simulink model "WheelSizing"  (R2023a)
settings: Solver=VariableStepAuto  StartTime=0.0  StopTime=6000  RelTol=1e-8
values from neighbouring files (symbols this model uses):
  euler_b_LVLH = [atan2(M(2,3),M(3,3)); -asin(M(1,3)); atan2(M(1,2),M(1,1))]    [A421_FinalProj_MainScript.m]    (also in WheelSizing_Script.m)
  I_ReactionWheels = J.normal + (2 * It + Is + 2 * mw) * eye(3)    [WheelSizing_Script.m]
  kd = 2 * zeta * wn .* J.normal    [WheelSizing_Script.m]
  kp = wn^2 * 2 .* J.normal    [WheelSizing_Script.m]
  qc = [0;0;0;1]    [WheelSizing_Script.m]
  r_ECI = Qperi2geo*r_PF    [WheelSizing_Script.m]
  rv_initial = [r_ECI;v_ECI]    [A421_FinalProj_MainScript.m]    (also in WheelSizing_Script.m)
  sun_ECI = [1; 0; 0]    [WheelSizing_Script.m]
  surfaceProperties = [Areas cps normals]    [WheelSizing_Script.m]
  v_ECI = Qperi2geo*v_PF    [WheelSizing_Script.m]
undefined symbols (not defined in the file or in its folder): J, normal
settings Model: Creator=jself  LastModifiedBy=willb
settings DebuggingCC: UnconnectedInputMsg=warning  UnconnectedOutputMsg=warning  UnconnectedLineMsg=warning
settings ModelReferenceCC: EnableRefExpFcnMdlSchedulingChecks=on
settings RTWCC: DLArmComputeVersion=19.05

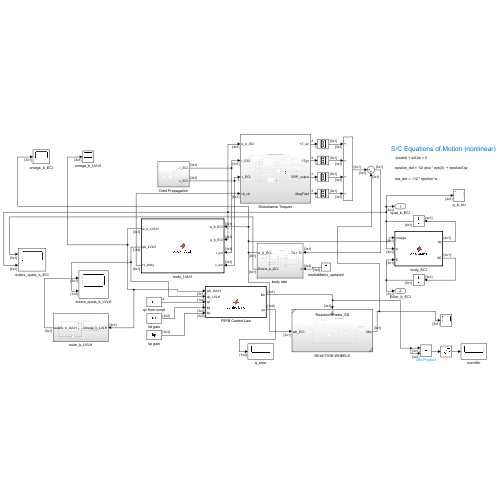
[thumbnail: Simulink's stored preview of the top-level diagram]
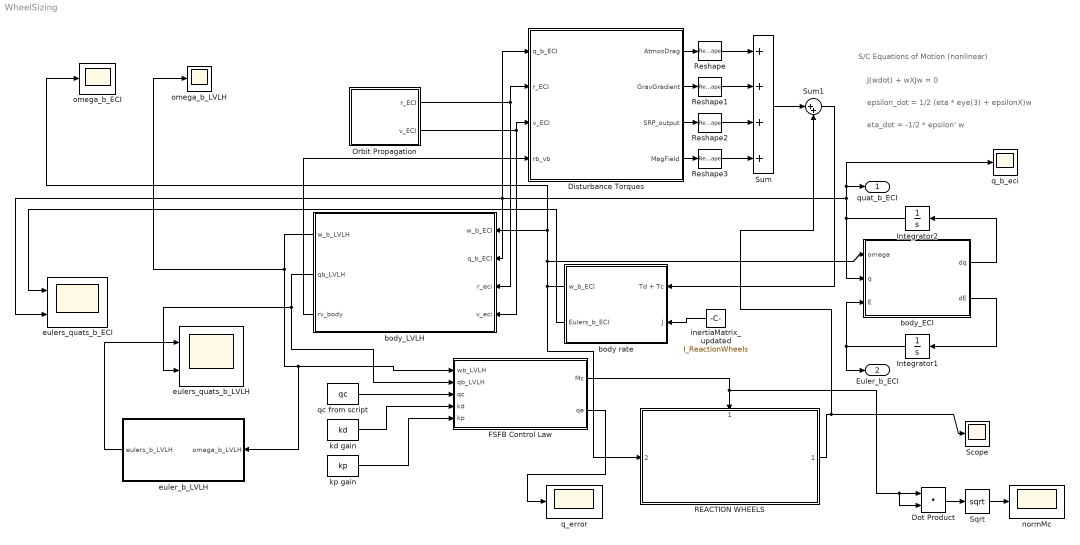
== system WheelSizing ==
  note: eta_dot = -1/2 * epsilon' w
  note: epsilon_dot = 1/2 (eta * eye(3) + epsilonX)w
  note: J(wdot) + wXJw = 0
  note: S/C Equations of Motion (nonlinear)
  Disturbance Torques : Subsystem
  Dot Product : DotProduct  OutDataTypeStr=Inherit: Inherit via internal rule
  FSFB Control Law : MATLAB Function  TreatAsAtomicUnit=on
  Integrator1 : Integrator  InitialCondition=normal.state(4:6)
  Integrator2 : Integrator  InitialCondition=normal.state(7:10)
  Orbit Propagation : Subsystem
  REACTION WHEELS : Subsystem  ReferencedSubsystem=ReactionWheels_SS
      settings: PortSchema="{\"entries\":[{\"content\":{\"sides\":[{\"content\":{\"connectorIds\":[\"In2\"]},\"type\":\"ConnectorPlacement.EquallySpacedRectSide\",\"uuid\":\"17b22d00-74c7-41dc-9281-1170939ab431\"},{\"content\":{\"connectorIds\":[\"Out1\"],\"side\":\"RIGHT\"},\"type\":\"ConnectorPlacement.EquallySpacedRectSide\",\"uuid\":\"47f34f04-9630-46fb-894e-c63a456fb1f8\"},{\"content\":{\"connectorIds\":[\"In1\"],\"side\":\"TOP\"},\"type\":\"ConnectorPlacement.EquallySpacedRectSide\",\"uuid\":\"0e15db1d-4c6b-4e54-83e4-cf923cd0db41\"}]},\"type\":\"ConnectorPlacement.EquallySpacedConnector\",\"uuid\":\"f035ae7b-0a11-467c-88f1-219b3350dd2e\"}],\"packageUris\":[\"http://schema.mathworks.com/mf0/Connector/R2020b\"],\"version\":\"1.0\"}"
  Reshape{,1..3} (4 alike) : Reshape  OutputDimensionality=Column vector (2-D)
  Scope : Scope
  Sqrt : Sqrt
  Sum : Sum  Inputs=++++
  Sum1 : Sum  Inputs=|++
  "body rate " : Subsystem
  body_ECI : MATLAB Function  TreatAsAtomicUnit=on
  body_LVLH : MATLAB Function  TreatAsAtomicUnit=on
  euler_b_LVLH : Subsystem
  eulers_quats_b_ECI : Scope  NumInputPorts=2
  eulers_quats_b_LVLH : Scope  NumInputPorts=2
  inertiaMatrix_updated : Constant  Value=I_ReactionWheels
  kd gain : Constant  Value=kd
  kp gain : Constant  Value=kp
  normMc : Scope
  omega_b_ECI : Scope
  omega_b_LVLH : Scope
  q_b_eci : Scope
  q_error : Scope
  qc from script : Constant  Value=qc
  quat_b_ECI : Outport  PortDimensions=[4 1]
  Euler_b_ECI : Outport  Port=2  PortDimensions=[3 1]
  wires:
  inertiaMatrix_updated/1 -> "body rate "/2(J)
  Disturbance Torques/1(AtmosDrag) -> Reshape/1
  Disturbance Torques/3(SRP_output) -> Reshape2/1
  body_LVLH/1(w_b_LVLH) -> omega_b_LVLH/1, euler_b_LVLH/1(omega_b_LVLH), FSFB Control Law/1(wb_LVLH)
  Orbit Propagation/1(r_ECI) -> body_LVLH/3(r_eci), Disturbance Torques/2(r_ECI)
  Orbit Propagation/2(v_ECI) -> Disturbance Torques/3(v_ECI), body_LVLH/4(v_eci)
  Sum1/1 -> "body rate "/1(Td + Tc)
  body_ECI/2(dE) -> Integrator1/1
  Integrator1/1 -> Euler_b_ECI/1, body_ECI/3(E)
  body_ECI/1(dq) -> Integrator2/1
  "body rate "/1(w_b_ECI) -> REACTION WHEELS/2, body_LVLH/1(w_b_ECI), omega_b_ECI/1, body_ECI/1(omega)
  kp gain/1 -> FSFB Control Law/5(kp)
  kd gain/1 -> FSFB Control Law/4(kd)
  qc from script/1 -> FSFB Control Law/3(qc)
  body_LVLH/2(qb_LVLH) -> eulers_quats_b_LVLH/2, FSFB Control Law/2(qb_LVLH)
  Integrator2/1 -> Disturbance Torques/1(q_b_ECI), eulers_quats_b_ECI/2, body_LVLH/2(q_b_ECI), q_b_eci/1, quat_b_ECI/1, body_ECI/2(q)
  body_LVLH/3(rv_body) -> Disturbance Torques/4(rb_vb)
  FSFB Control Law/2(qe) -> q_error/1
  FSFB Control Law/1(Mc) -> Dot Product/2, Dot Product/1, REACTION WHEELS/1
  Sum/1 -> Sum1/1
  Reshape/1 -> Sum/1
  Disturbance Torques/4(MagField) -> Reshape3/1
  Reshape3/1 -> Sum/4
  Reshape2/1 -> Sum/3
  Disturbance Torques/2(GravGradient) -> Reshape1/1
  Reshape1/1 -> Sum/2
  "body rate "/2(Eulers_b_ECI) -> eulers_quats_b_ECI/1
  euler_b_LVLH/1(eulers_b_LVLH) -> eulers_quats_b_LVLH/1
  REACTION WHEELS/1 -> Sum1/2, Scope/1
  Sqrt/1 -> normMc/1
  Dot Product/1 -> Sqrt/1

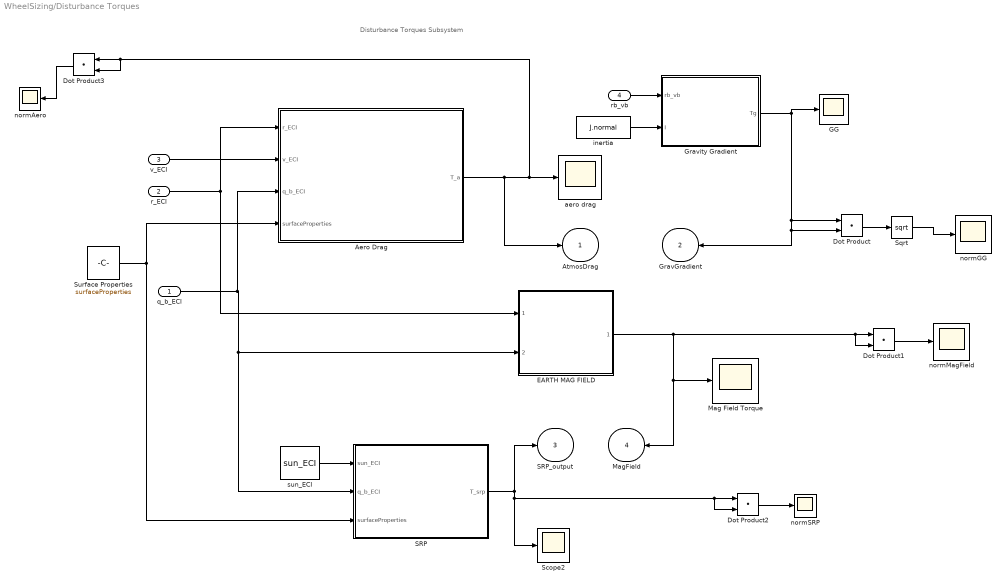
== system WheelSizing/Disturbance Torques ==
  note: Disturbance Torques Subsystem
  q_b_ECI : Inport  PortDimensions=[4 1]
  r_ECI : Inport  Port=2
  v_ECI : Inport  Port=3  PortDimensions=3
  rb_vb : Inport  Port=4
  Aero Drag : MATLAB Function  TreatAsAtomicUnit=on
  Dot Product{,1..3} (4 alike) : DotProduct  OutDataTypeStr=Inherit: Inherit via internal rule
  EARTH MAG FIELD : Subsystem  ReferencedSubsystem=EarthMagneticField_SS
  GG : Scope
  Gravity Gradient : MATLAB Function  TreatAsAtomicUnit=on
  Mag Field Torque : Scope
  SRP : MATLAB Function  TreatAsAtomicUnit=on
  Scope2 : Scope
  Sqrt : Sqrt
  Surface Properties : Constant  Value=surfaceProperties
  aero drag : Scope
  inertia : Constant  Value=J.normal
  normAero : Scope
  normGG : Scope
  normMagField : Scope
  normSRP : Scope
  sun_ECI : Constant  Value=sun_ECI
  AtmosDrag : Outport
  GravGradient : Outport  Port=2
  SRP_output : Outport  Port=3
  MagField : Outport  Port=4
  wires:
  Gravity Gradient/1(Tg) -> GG/1, Dot Product/1, Dot Product/2, GravGradient/1
  SRP/1(T_srp) -> Scope2/1, Dot Product2/2, Dot Product2/1, SRP_output/1
  Aero Drag/1(T_a) -> Dot Product3/2, Dot Product3/1, aero drag/1, AtmosDrag/1
  sun_ECI/1 -> SRP/1(sun_ECI)
  v_ECI/1 -> Aero Drag/2(v_ECI)
  q_b_ECI/1 -> SRP/2(q_b_ECI), EARTH MAG FIELD/2, Aero Drag/3(q_b_ECI)
  r_ECI/1 -> EARTH MAG FIELD/1, Aero Drag/1(r_ECI)
  EARTH MAG FIELD/1 -> MagField/1, Mag Field Torque/1, Dot Product1/2, Dot Product1/1
  Surface Properties/1 -> SRP/3(surfaceProperties), Aero Drag/4(surfaceProperties)
  rb_vb/1 -> Gravity Gradient/1(rb_vb)
  inertia/1 -> Gravity Gradient/2(I)
  Dot Product/1 -> Sqrt/1
  Sqrt/1 -> normGG/1
  Dot Product1/1 -> normMagField/1
  Dot Product2/1 -> normSRP/1
  Dot Product3/1 -> normAero/1

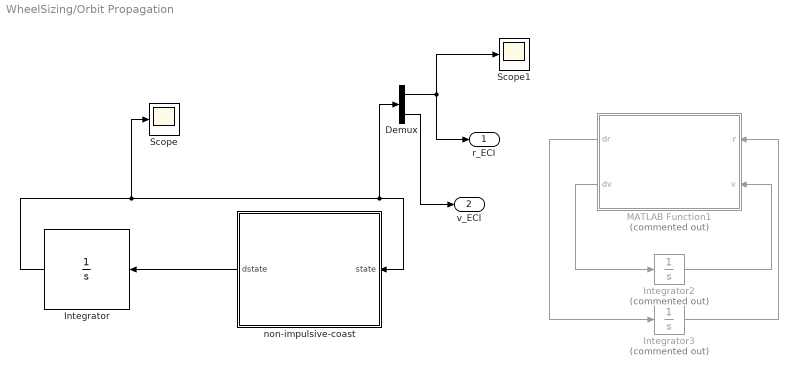
== system WheelSizing/Orbit Propagation ==
  Demux : Demux  Outputs=2
  Integrator : Integrator  InitialCondition=rv_initial
  Integrator2 : Integrator  Commented=on  InitialCondition=r_ECI
  Integrator3 : Integrator  Commented=on  InitialCondition=v_ECI
  MATLAB Function1 : MATLAB Function  Commented=on  TreatAsAtomicUnit=on
  Scope : Scope
  Scope1 : Scope
  non-impulsive-coast : MATLAB Function  TreatAsAtomicUnit=on
  r_ECI : Outport  PortDimensions=[3 1]  VectorParamsAs1DForOutWhenUnconnected=off
  v_ECI : Outport  Port=2  PortDimensions=[3 1]  VectorParamsAs1DForOutWhenUnconnected=off
  wires:
  Integrator2/1 -> MATLAB Function1/2(v)
  MATLAB Function1/1(dr) -> Integrator3/1
  MATLAB Function1/2(dv) -> Integrator2/1
  Integrator3/1 -> MATLAB Function1/1(r)
  non-impulsive-coast/1(dstate) -> Integrator/1
  Integrator/1 -> Scope/1, Demux/1, non-impulsive-coast/1(state)
  Demux/1 -> Scope1/1, r_ECI/1
  Demux/2 -> v_ECI/1

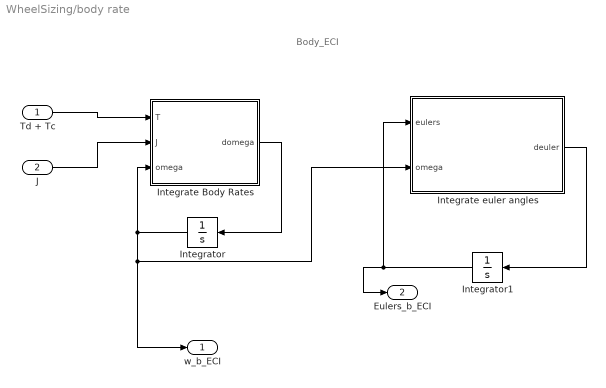
== system WheelSizing/body rate  ==
  note: Body_ECI
  Td + Tc : Inport
  J : Inport  Port=2
  Integrate Body Rates : MATLAB Function  TreatAsAtomicUnit=on
  Integrate euler angles : MATLAB Function  TreatAsAtomicUnit=on
  Integrator : Integrator  InitialCondition=normal.state(1:3)
  Integrator1 : Integrator  InitialCondition=normal.state(4:6)
  w_b_ECI : Outport  PortDimensions=[3 1]
  Eulers_b_ECI : Outport  Port=2
  wires:
  J/1 -> Integrate Body Rates/2(J)
  Td + Tc/1 -> Integrate Body Rates/1(T)
  Integrate Body Rates/1(domega) -> Integrator/1
  Integrator/1 -> Integrate euler angles/2(omega), w_b_ECI/1, Integrate Body Rates/3(omega)
  Integrate euler angles/1(deuler) -> Integrator1/1
  Integrator1/1 -> Eulers_b_ECI/1, Integrate euler angles/1(eulers)

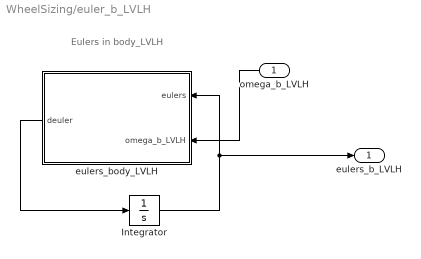
== system WheelSizing/euler_b_LVLH ==
  note: Eulers in body_LVLH
  omega_b_LVLH : Inport
  Integrator : Integrator  InitialCondition=euler_b_LVLH
  eulers_body_LVLH : MATLAB Function  TreatAsAtomicUnit=on
  eulers_b_LVLH : Outport
  wires:
  eulers_body_LVLH/1(deuler) -> Integrator/1
  Integrator/1 -> eulers_b_LVLH/1, eulers_body_LVLH/1(eulers)
  omega_b_LVLH/1 -> eulers_body_LVLH/2(omega_b_LVLH)

== matlab function WheelSizing/Disturbance Torques/Aero Drag ==
  data: r_ECI input; v_ECI input; T_a output; q_b_ECI input; surfaceProperties input
function T_a = aero_drag_torque(r_ECI, v_ECI, q_b_ECI, surfaceProperties) 


q_b_ECI = q_b_ECI'; 
q_b_ECI = [q_b_ECI(4), q_b_ECI(1), q_b_ECI(2), q_b_ECI(3)]; 
v_b = quat2rotm(q_b_ECI)*v_ECI;
Cd = 2.1;
Re = 6378.137;

rho_0 = 3.614e-14;
H = 88.667;
h_0 = 700;
density = rho_0*exp(-(norm(r_ECI) - Re - h_0)/H);
T_a = zeros([3,1]);

for i = 1:length(surfaceProperties)
    A = surfaceProperties(i,1);
    cp = surfaceProperties(i,2:4);
    n = surfaceProperties(i,5:7);
    wet = n*v_b/norm(v_b);
    if wet > 0
        A_wet = A*wet;
        v_b_hat = v_b/norm(v_b);
        F_a = -1/2*density*(norm(v_ECI)*1000)^2*Cd*A_wet*v_b_hat;
        T_a = T_a + cross(cp', F_a);
    end
end

== matlab function WheelSizing/FSFB Control Law ==
  data: wb_LVLH input; qb_LVLH input; qc input; Mc output; kd input; kp input; qe output
% this is JUSTIN'S gain selection code from an old assignment

function [Mc,qe]  = controlLaw(wb_LVLH, qb_LVLH, qc, kd, kp)

% Torque output goes to equations of motion
% epsilon error only ouputting to verify that it converges to 0. 

qc = [qc(4),qc(1),qc(2),qc(3)]; % ROW; ETA FIRST

% MODIFYING INPUTS; quaternion only
% 1. ROW VECTOR
% 2. ETA FIRST, THEN EPSILON for all MATLAB quat functions

q = qb_LVLH; % row; ETA FIRST 
w = wb_LVLH; 

% We give up and create our functions...
qe = quatMult(quatConj(qc),q);
% out == eta first; row
% qe = [qe(4),qe(1),qe(2),qe(3)]; % now ETA IS FIRST

Epsilon_error = qe(2:4); % row; eta first.

% Control law
Mc = -kp*Epsilon_error' - kd*w;
 
end

== matlab function WheelSizing/body rate /Integrate euler angles ==
  data: eulers input; deuler output; omega input
function deuler = euler_rates(eulers,omega)

% Euler Angles
phi = eulers(1);
theta = eulers(2);
psi = eulers(3);

deuler = cos(theta)^(-1) * [   cos(theta)      sin(phi)*sin(theta)     cos(phi)*sin(theta); 
                                0               cos(phi)*cos(theta)     -sin(phi)*cos(theta);
                                0               sin(phi)                 cos(phi)           ] * omega;

== matlab function WheelSizing/body_LVLH ==
  data: w_b_ECI input; q_b_ECI input; r_eci input; v_eci input; w_b_LVLH output; qb_LVLH output; rv_body output
function [w_b_LVLH, qb_LVLH, rv_body] = body_LVLH(w_b_ECI, q_b_ECI, r_eci, v_eci)

% ASSUME ETA COMES IN FIRST
% epsilon_ECI = q_b_ECI(2:4); 
% eta_ECI = q_b_ECI(1); 
epsilon_ECI = q_b_ECI(1:3); 
eta_ECI = q_b_ECI(4);


[Cb_ECI] = quat2rotationmatrix(epsilon_ECI,eta_ECI); 

w_LVLH_ECI = (cross(r_eci,v_eci))/(norm(r_eci)^2);  
w_b_LVLH = w_b_ECI - Cb_ECI*w_LVLH_ECI; 

% ECI to LVLH for getting q_b_LVLH 
rmag_eci = norm(r_eci);                                                     
h_eci = cross(r_eci,v_eci);
hmag_eci = norm(h_eci);

% ECI to LVLH
z = -r_eci/rmag_eci;
y = -h_eci/hmag_eci;
x = cross(y,z);
C_LVLH_ECI = [x'; y'; z'];

% Get Cb_LVLH
Cb_LVLH = Cb_ECI * C_LVLH_ECI'; 

% Get qb_LVLH 
qb_LVLH = C2quat_altVersion(Cb_LVLH); % ROW VECTOR; eta first 
%qb_LVLH = C2quat(Cb_LVLH); %eta first

rv_body = [Cb_ECI * r_eci; Cb_ECI * v_eci]; 


end

== matlab function WheelSizing/euler_b_LVLH/eulers_body_LVLH ==
  data: eulers input; deuler output; omega_b_LVLH input
function deuler = euler_rates(eulers,omega_b_LVLH)

% Euler Angles

phi = eulers(1);
theta = eulers(2);
psi = eulers(3);

deuler = cos(theta)^(-1) * [   cos(theta)      sin(phi)*sin(theta)     cos(phi)*sin(theta); 
                                0               cos(phi)*cos(theta)     -sin(phi)*cos(theta);
                                0               sin(phi)                 cos(phi)           ] * omega_b_LVLH;

== matlab function WheelSizing/Orbit Propagation/MATLAB Function1 ==
  data: r input; dr output; v input; dv output
function [dr,dv] = orbitalDynamic(r,v)

mu = 398600; 

dr = v; 
dv = -mu*r/norm(r); 

end

== matlab function WheelSizing/body rate /Integrate Body Rates ==
  data: T input; domega output; J input; omega input
function domega  = dynamics(T, J, omega)

domega = J\(T - cross(omega, J*omega)); 

end

== matlab function WheelSizing/Orbit Propagation/non-impulsive-coast ==
  data: state input; dstate output
function dstate = non_impulsive_COAST(state)
%{ 

*FOR COAST PHASE ONLY*

**This function assumes that thrust is exactly parallel to initial velocity
direction.

This function is for numerical integration (i.e., plug into ode45).
NOTE: only use this function for the BURN PHASE of the non-impulsive
maneuver. For the BURN phase, use "non_impulsive_BURN"

INPUTS: 
    INITIAL CONDITIONS
    state vector(1:3) = position (rx,ry,rz)
    state vector(4:6) = velocity (vx,vy,vz)

OUTPUT: New state vector after integration.
%%%%%%%%%%%%%%%%%%%%%%%%%%%%%%%%%%%%%%%%%%%%%%%%%
Justin Self, Cal Poly, Fall 2022; Introduction to Orbital Mechanics.
%%%%%%%%%%%%%%%%%%%%%%%%%%%%%%%%%%%%%%%%%%%%%%%%%
%}

mu = 398600;

rx = state(1);
ry = state(2);
rz = state(3);
vx = state(4);
vy = state(5);
vz = state(6);

r_vect = [rx ry rz];
r = norm(r_vect);

v_vect = [vx vy vz];
v = norm(v_vect);

xdot = vx;
ydot = vy;
zdot = vz;
xddot = (-mu*rx)/(r^3);
yddot = (-mu*ry)/(r^3);
zddot = (-mu*rz)/(r^3);

dstate = [xdot; ydot; zdot; xddot; yddot; zddot];

% rState = dstate(1:3);
% vState = dstate(4:6);

end

== matlab function WheelSizing/body_ECI ==
  data: omega input; dq output; q input; E input; dE output
function [dq,dE] = kinematics(omega, q, E)


% unpack quaternion
% epsilon = q(1:3,1);
% eta = q(4,1);
% depsilon = 1/2*(eta*eye(3) + vect2cross(epsilon))*omega;
% deta = -1/2*epsilon'*omega;
% dq = [depsilon; deta];

epx = q(1);
epy = q(2);
epz = q(3);
eta = q(4);
epsilon = [epx; epy; epz];
epsilon_cross = [   0       -epz     epy;
                    epz     0        -epx;
                    -epy    epx      0    ];

% Derivatives of epsilon and eta
depsilon = 0.5 * (eta*eye(3) + epsilon_cross) * omega;
deta = -0.5 * epsilon' * omega;
dq = [depsilon(1); depsilon(2); depsilon(3); deta]; % ETA LAST

% Euler Angle 
LBI = 1/cos(E(2))*[cos(E(2)) sin(E(1))*sin(E(2))  cos(E(1))*sin(E(2));
                   0         cos(E(1))*cos(E(2)) -sin(E(1))*cos(E(2));
                   0         sin(E(1))            cos(E(1))];
dE = LBI*omega;

end

== matlab function WheelSizing/Disturbance Torques/SRP ==
  data: sun_ECI input; T_srp output; q_b_ECI input; surfaceProperties input
function T_srp  = SPR_torque(sun_ECI, q_b_ECI, surfaceProperties)

p_sun = 4.5e-6; %N/m
q_b_ECI = q_b_ECI'; 
q_b_ECI = [q_b_ECI(4), q_b_ECI(1), q_b_ECI(2), q_b_ECI(3)]; 

sun_b = quat2rotm(q_b_ECI) * sun_ECI;
T_srp = zeros([3,1]);
%rho_sum = zeros([3,1]);
% Solar Radiation Pressure
for i = 1:length(surfaceProperties)
    A = surfaceProperties(i,1);
    cp = surfaceProperties(i,2:4);
    n = surfaceProperties(i,5:7);
    wet = n*sun_b/norm(sun_b);
    if wet > 0
        A_wet = A*wet;
        F_srp = p_sun*A_wet*sun_b;
        T_srp = T_srp + cross(cp', F_srp);
        %rho_sum = rho_sum + rho';
    end
end

== matlab function WheelSizing/Disturbance Torques/Gravity Gradient ==
  data: rb_vb input; Tg output; I input
% function T_gg = gg_torque(r_ECI, q_b_ECI, J)
% 
% mu = 398600;
% 
% % R in body
% r_b = quat2rotm(q_b_ECI)*r_ECI;
% % Gravity Gradient Torque
% T_gg = 3*mu/norm(r_b)^5 * vect2cross(r_b)*J*(r_b);  

function Tg = gravgradient(rb_vb,I)

mu = 398600;
rb = rb_vb(1:3);
rb_cross = [     0       -rb(3)     rb(2);
                rb(3)    0         -rb(1);
               -rb(2)    rb(1)       0   ];
Tg = ( (3*mu) / (norm(rb)^5) ) * (rb_cross * I * rb); 

% 3x1; good
end
